simulink model "controllerModel"  (R2020b)
settings: Solver=VariableStepAuto  StartTime=0.0  StopTime=10  MaxStep=1e-3  RelTol=1e-3
model workspace (MAT data in the model file):
  TrqICMax = 250
  TrqMGUMax = 50
  TrqMax = 300
  brkTrqMGU = 25
  brkTrqMax = 100
settings Model: Creator=mordi  LastModifiedBy=mordi

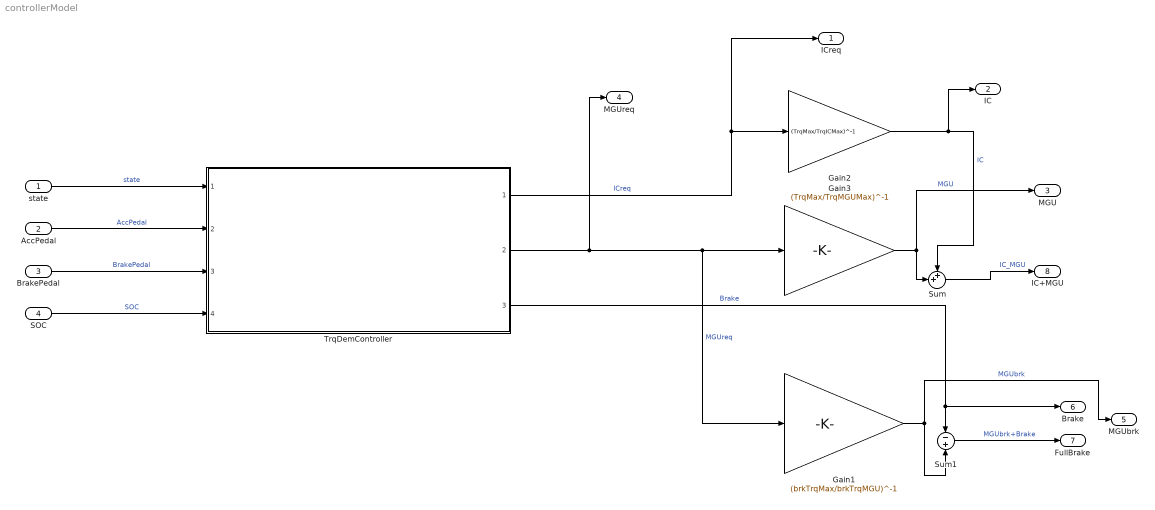
== system controllerModel ==
  state : Inport
  AccPedal : Inport  Port=2
  BrakePedal : Inport  Port=3
  SOC : Inport  Port=4
  Gain1 : Gain  Gain=(brkTrqMax/brkTrqMGU)^-1
  Gain2 : Gain  Gain=(TrqMax/TrqICMax)^-1
  Gain3 : Gain  Gain=(TrqMax/TrqMGUMax)^-1
  Sum : Sum  Inputs=++|
  Sum1 : Sum  Inputs=-+
  TrqDemController : Subsystem  ReferencedSubsystem=TrqDemController
  ICreq : Outport
  IC : Outport  Port=2
  MGU : Outport  Port=3
  MGUreq : Outport  Port=4
  MGUbrk : Outport  Port=5
  Brake : Outport  Port=6
  FullBrake : Outport  Port=7
  IC+MGU : Outport  Port=8
  wires:
  Sum1/1 -> FullBrake/1  "MGUbrk+Brake"
  BrakePedal/1 -> TrqDemController/3  "BrakePedal"
  state/1 -> TrqDemController/1  "state"
  SOC/1 -> TrqDemController/4  "SOC"
  AccPedal/1 -> TrqDemController/2  "AccPedal"
  Gain1/1 -> MGUbrk/1, Sum1/2  "MGUbrk"
  TrqDemController/1 -> ICreq/1, Gain2/1  "ICreq"
  TrqDemController/3 -> Brake/1, Sum1/1  "Brake"
  Gain2/1 -> IC/1, Sum/1  "IC"
  Gain3/1 -> Sum/2, MGU/1  "MGU"
  TrqDemController/2 -> MGUreq/1, Gain1/1, Gain3/1  "MGUreq"
  Sum/1 -> IC+MGU/1  "IC_MGU"
